simulink model "DR_Screening_Resource_Model"  (R2026a)
settings: Solver=FixedStepDiscrete  StopTime=480  FixedStep=1
settings Model: Creator=krish  LastModifiedBy=krish

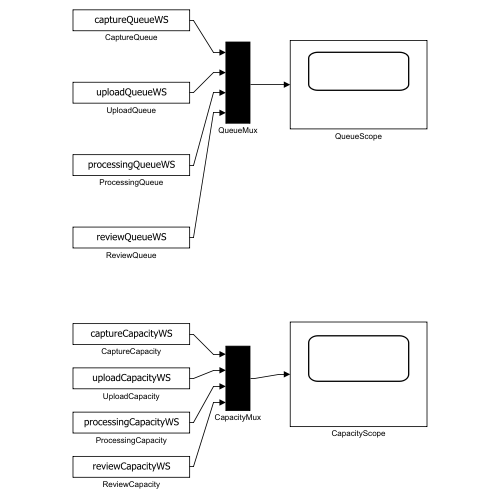
[thumbnail: Simulink's stored preview of the top-level diagram]
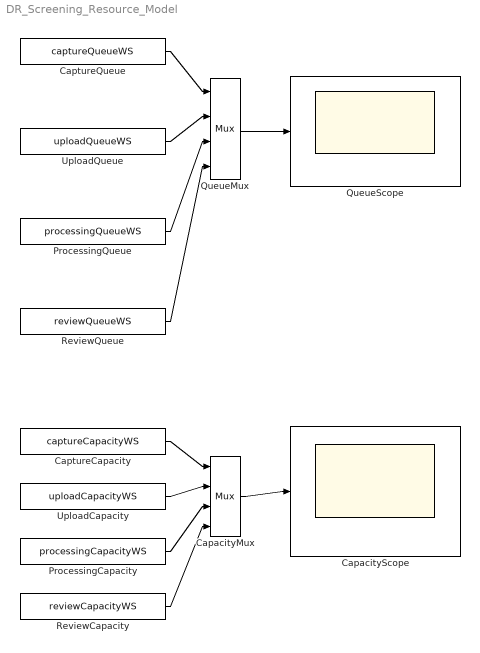
== system DR_Screening_Resource_Model ==
  CapacityMux : Mux
  CapacityScope : Scope
  CaptureCapacity : FromWorkspace  VariableName=captureCapacityWS
  CaptureQueue : FromWorkspace  VariableName=captureQueueWS
  ProcessingCapacity : FromWorkspace  VariableName=processingCapacityWS
  ProcessingQueue : FromWorkspace  VariableName=processingQueueWS
  QueueMux : Mux
  QueueScope : Scope
  ReviewCapacity : FromWorkspace  VariableName=reviewCapacityWS
  ReviewQueue : FromWorkspace  VariableName=reviewQueueWS
  UploadCapacity : FromWorkspace  VariableName=uploadCapacityWS
  UploadQueue : FromWorkspace  VariableName=uploadQueueWS
  wires:
  CaptureQueue/1 -> QueueMux/1
  UploadQueue/1 -> QueueMux/2
  ProcessingQueue/1 -> QueueMux/3
  ReviewQueue/1 -> QueueMux/4
  QueueMux/1 -> QueueScope/1
  CaptureCapacity/1 -> CapacityMux/1
  UploadCapacity/1 -> CapacityMux/2
  ProcessingCapacity/1 -> CapacityMux/3
  ReviewCapacity/1 -> CapacityMux/4
  CapacityMux/1 -> CapacityScope/1
